simulink model "AP_DiffEQs"  (Simulink 8.4)
settings: Solver=ode45  StartTime=0.0  StopTime=10.0  RelTol=1e-3
settings Model: Creator=Monica  LastModifiedBy=Monica
settings DataIOCC: SignalLoggingSaveFormat=Dataset
settings OptimizationCC: ExpressionDepthLimit=128
settings DebuggingCC: UnderspecifiedInitializationDetection=Simplified  MergeDetectMultiDrivingBlocksExec=error  FcnCallInpInsideContextMsg=EnableAllAsError  StateNameClashWarn=none
settings GRTTargetCC: CombineOutputUpdateFcns=on  GRTInterface=off

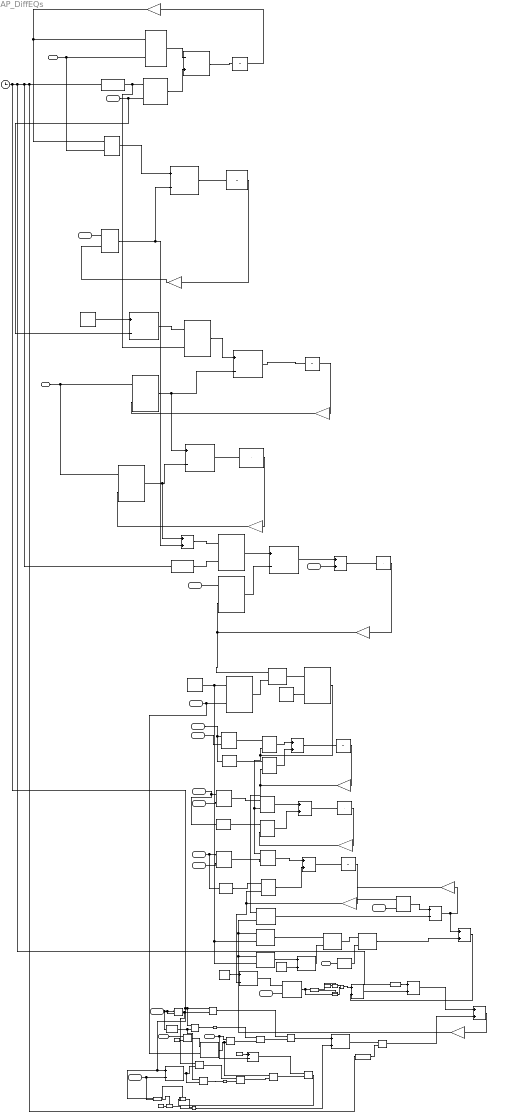
== system AP_DiffEQs ==
  note: 0
  note: false
  note: true
  note: t
  note: d
  note: Q_sub_2
  note: Q_sub_2
  note: Q_sub_1
  note: Q_sub_1
  note: Q_sub_1
  note: Q_sub_1
  note: -F_sub_01*(Q_sub_1/V)/(1+Q_sub_1/V)-x_sub_1*Q_sub_1+k_sub_12*Q_sub_2+EGP_0(1-x_sub_3)+f_sub_g+U_sub_m
  note: (U_sub_m1+U_sub_m2)*f_sub_m=U_sub_m
  note: f_sub_m
  note: t
  note: (U_sub_m1 + U_sub_m2)
  note: U_sub_m2
  note: (t-d)*(k_sub_m^2)*(exp((-k_sub_m)*(t-d)))*((CHO*5551)/w)*(1-p_sub_m)
  note: (1-p_sub_m)
  note: (1-p_sub_m)
  note: p_sub_m
  note: 1
  note: (t-d)*(k_sub_m^2)*(exp((-k_sub_m)*(t-d)))*((CHO*5551)/w)
  note: 0
  note: (t-d)*(k_sub_m^2)(*exp((-k_sub_m)*(t-d)))
  note: (t-d)*(k_sub_m^2)*(exp((-k_sub_m)*(t-d)))
  note: exp((-k_sub_m)*(t-d))
  note: (-k_sub_m)*(t-d)
  note: (t-d)
  note: -k_sub_m
  note: k_sub_m^2)
  note: (t-d)*(k_sub_m^2)
  note: (t-d)
  note: d
  note: t
  note: ((k_sub_m^2)*t)*exp(-k_sub_m*t)*((CHO*5551)/w)*p_sub_m
  note: exp(-k_sub_m*t)*((CHO*5551)/w)*p_sub_m
  note: ((k_sub_m^2)*t)
  note: ((CHO*5551)/w)*p_sub_m
  note: (CHO*5551)/w
  note: CHO*5551
  note: 5551
  note: CHO
  note: (k_sub_m^2*t)
  note: exp(-k_sub_m*t)
  note: -k_sub_m*t
  note: t
  note: -k_sub_m
  note: t
  note: k_sub_m^2
  note: k_sub_m
  note: k_sub_m
  note: -F_sub_01*(Q_sub_1/V)/(1+Q_sub_1/V)-x_sub_1*Q_sub_1+k_sub_12*Q_sub_2+EGP_0(1-x_sub_3)+f_sub_g
  note: -F_sub_01*(Q_sub_1/V)/(1+Q_sub_1/V)-x_sub_1*Q_sub_1+k_sub_12*Q_sub_2+EGP_0(1-x_sub_3)
  note: -F_sub_01*(Q_sub_1/V)/(1+Q_sub_1/V)-x_sub_1*Q_sub_1+k_sub_12*Q_sub_2
  note: EGP_0*(1-x_sub_3)
  note: 1
  note: EGP_0
  note: x_sub_3
  note: 1-x_sub_3
  note: -x_sub_1*Q_sub_1+k_sub_12*Q_sub_2
  note: x_sub_1*Q_sub_1
  note: k_sub_12*Q_sub_2
  note: -F_sub_01*(Q_sub_1/V)/(1+Q_sub_1/V)
  note: (Q_sub_1/V)/(1+Q_sub1/V)
  note: Q_sub_1/V + 1
  note: Q_sub_1/V
  note: x_sub_1
  note: V
  note: V
  note: Q_sub_1/V
  note: -F_sub_01
  note: F_sub_01
  note: x_sub_3
  note: -k_sub_a3*x_sub_3+k_sub_a3*S_sub_e*I_sub_p
  note: -k_sub_a3*x_sub_3
  note: k_sub_a3*S_sub_e*I_sub_p
  note: x_sub_3
  note: -k_sub_a3
  note: k_sub_a3*S_sub_e
  note: S_sub_e
  note: k_sub_a3
  note: k_sub_a3
  note: x_sub_2
  note: -k_sub_a2*x_sub_2+k_sub_a2*S_sub_d*I_sub_p
  note: -k_sub_a2*x_sub_2
  note: k_sub_a2*S_sub_d*I_sub_p
  note: k_sub_a2*S_sub_d
  note: I_sub_p
  note: -k_sub_a2
  note: k_sub_a2
  note: S_sub_d
  note: k_sub_a2
  note: x_sub_1
  note: -k_sub_a1
  note: -k_sub_a1*x_sub_1+k_sub_a1*S_sub_t*I_sub_p
  note: -k_sub_a1*x_sub_1
  note: I_sub_p
  note: k_sub_a1*S_sub_t*I_sub_p
  note: I_sub_p
  note: k_sub_a1
  note: S_sub_t
  note: k_sub_a1
  note: Q_sub_i/V_sub_i*w
  note: Q_sub_i
  note: w
  note: V_sub_i
  note: V_sub_i*w
  note: Q_sub_i
  note: ((Q_sub_is2*k_sub_is2+Q_sub_if2*k_sub_if)*I_sub_m)-Q_sub_i*k_sub_e+c_sub_i
  note: ((Q_sub_is2*k_sub_is2+Q_sub_if2*k_sub_if)*I_sub_m)-Q_subI*k_sub_e
  note: (Q_sub_is2*k_sub_is2+Q_sub_if2*k_sub_if)*I_sub_m
  note: Q_sub_i*k_sub_e
  note: I_sub_m
  note: Q_sub_is2*k_sub_is2+Q_sub_if2*k_sub_if
  note: Q_sub_is2*k_sub_is2
  note: Q_sub_if2*k_sub_if
  note: Q_sub_if1*k_sub_if-Q_sub_if2*k_sub_if
  note: Q_sub_if1*k_sub_if
  note: Q_sub_if2*k_sub_if
  note: Q_sub_if2
  note: k_sub_if
  note: Q_sub_if1
  note: (u_sub_i(t))*(1-p_sub_i)-Q_sub_i1f*k_sub_if
  note: Q_sub_if1*k_sub_if
  note: (u_sub_i(t))*(1-p_sub_i)
  note: u_sub_i(t)
  note: 1
  note: p_sub_i
  note: (1-p_sub_i)
  note: Q_sub_is1*k_sub_is1-Q_sub_is2*k_sub_is2
  note: Q_sub_is2*k_sub_is2
  note: Q_sub_is2
  note: Q_sub_is1*k_sub_is1
  note: k_sub_is1
  note: Q_sub_is1
  note: Q_sub_is1
  note: (u_sub_i(t)*p_sub_i)-(Q_sub_is1(t)*k_sub_is1)
  note: u_sub_i(t)*p_sub_i
  note: Q_sub_is1(t)*k_sub_is1
  p_sub_i : Inport
  "k_sub_is1 " : Inport  Port=2
  "k_sub_is2 " : Inport  Port=3
  k_sub_if : Inport  Port=4
  k_sub_e : Inport  Port=5
  c_sub_i : Inport  Port=6
  "w " : Inport  Port=7
  k_sub_a1 : Inport  Port=8
  S_sub_t : Inport  Port=9
  k_sub_a2 : Inport  Port=10
  S_sub_d : Inport  Port=11
  k_sub_a3 : Inport  Port=12
  S_sub_e : Inport  Port=13
  F_sub_01 : Inport  Port=14
  k_sub_12 : Inport  Port=15
  EGP_0 : Inport  Port=16
  k_sub_m : Inport  Port=17
  CHO : Inport  Port=18
  p_sub_m : Inport  Port=19
  d : Inport  Port=20
  " " : FunctionCaller  FunctionPrototype=u_sub_i = f(t)
  10^6 : Constant  Value=10^6
  Add{,1..5,8..10,13..14} (11 alike) : Sum
  Add{6..7,11..12} (4 alike) : Sum  Inputs=+-
  Clock : Clock
  Constant{,1..2,6} (4 alike) : Constant
  Constant3 : Constant  Value=0
  Constant4 : Constant  Value=5551
  Constant5 : Constant  Value=0
  Divide{,1..4} (5 alike) : Product  Inputs=*/
  Gain{,1..9} (10 alike) : Gain
  I_sub_m(t) : FunctionCaller  FunctionPrototype=I_sub_m = f(t)
  If : If  IfExpression=u1 >= 1
  If Action Subsystem : Subsystem  TreatAsAtomicUnit=on
  If Action Subsystem1 : Subsystem  TreatAsAtomicUnit=on
  If Action Subsystem2 : Subsystem  TreatAsAtomicUnit=on
  If Action Subsystem3 : Subsystem  TreatAsAtomicUnit=on
  Integrator{,1..7} (8 alike) : Integrator
  Math Function : Math  SaturateOnIntegerOverflow=on
  Math Function1 : Math  SaturateOnIntegerOverflow=on
  Merge : Merge
  Merge1 : Merge
  Product{,1..36} (37 alike) : Product
  Subtract : Sum  Inputs=-+
  Subtract{1..5} (5 alike) : Sum  Inputs=+-
  Subtract{6..10} (5 alike) : Sum  Inputs=-
  V_sub_i : Constant  Value=190
  f_sub_g : FunctionCaller  FunctionPrototype=f_sub_g = f(t)
  f_sub_m(t) : FunctionCaller  FunctionPrototype=f_sub_m = f(t)
  t-d : If  NumInputs=2  IfExpression=u1 > u2
  "u_sub_i(t) " : FunctionCaller  FunctionPrototype=u_sub_i = f(t)
  wires:
  Clock/1 -> Add11/1, t-d/1, Product26/1, Product25/1, f_sub_g/1, I_sub_m(t)/1, f_sub_m(t)/1, " "/1
  "k_sub_is1 "/1 -> Product2/2, Product/2
  " "/1 -> Product4/2, Product1/1
  p_sub_i/1 -> Subtract2/2, Product1/2
  Product/1 -> Subtract/1
  Product1/1 -> Subtract/2
  Subtract/1 -> Integrator/1
  Integrator/1 -> Gain/1
  Gain/1 -> Product2/1, Product/1
  Product2/1 -> Subtract1/1
  "k_sub_is2 "/1 -> Product3/1
  Product3/1 -> Add/2, Subtract1/2
  Subtract1/1 -> Integrator1/1
  Integrator1/1 -> Gain1/1
  Gain1/1 -> Product3/2
  Constant/1 -> Subtract2/1
  Subtract2/1 -> Product4/1
  k_sub_if/1 -> Product6/1, Product5/1
  Product5/1 -> Subtract3/2, Subtract4/1
  Product4/1 -> Subtract3/1
  Subtract3/1 -> Integrator2/1
  Integrator2/1 -> Gain2/1
  Gain2/1 -> Product5/2
  Product6/1 -> Add/1, Subtract4/2
  Subtract4/1 -> Integrator3/1
  Integrator3/1 -> Gain3/1
  Gain3/1 -> Product6/2
  Add/1 -> Product7/1
  I_sub_m(t)/1 -> Product7/2
  Product7/1 -> Subtract5/1
  k_sub_e/1 -> Product8/1
  Product8/1 -> Subtract5/2
  Subtract5/1 -> Add1/1
  c_sub_i/1 -> Add1/2
  Add1/1 -> Integrator4/1
  Integrator4/1 -> Gain4/1
  Gain4/1 -> Divide/1, Product8/2
  Product9/1 -> Divide/2
  V_sub_i/1 -> Divide1/2, Divide2/2, Product9/1
  "w "/1 -> Divide4/2, Product9/2
  Divide/1 -> Product10/1
  10^6/1 -> Product10/2
  k_sub_a1/1 -> Subtract6/1, Product11/1
  S_sub_t/1 -> Product11/2
  Product11/1 -> Product12/1
  Subtract6/1 -> Product13/1
  Product10/1 -> Product18/1, Product16/2, Product12/2
  Product12/1 -> Add2/1
  Product13/1 -> Add2/2
  Add2/1 -> Integrator5/1
  Integrator5/1 -> Gain5/1
  Gain5/1 -> Product13/2, Product20/1
  k_sub_a2/1 -> Subtract7/1, Product14/1
  S_sub_d/1 -> Product14/2
  Subtract7/1 -> Product15/1
  Product14/1 -> Product16/1
  Product16/1 -> Add3/1
  Product15/1 -> Add3/2
  Add3/1 -> Integrator6/1
  Integrator6/1 -> Gain6/1
  Gain6/1 -> Product15/2
  k_sub_a3/1 -> Subtract8/1, Product17/1
  S_sub_e/1 -> Product17/2
  Product17/1 -> Product18/2
  Subtract8/1 -> Product19/1
  Product18/1 -> Add4/1
  Product19/1 -> Add4/2
  Integrator7/1 -> Gain7/1
  Add4/1 -> Integrator7/1
  Gain7/1 -> Product19/2, Add7/2
  Divide2/1 -> Add5/1
  Constant1/1 -> Add5/2
  Add5/1 -> Divide3/2
  Divide1/1 -> Divide3/1
  Divide3/1 -> Product21/1
  F_sub_01/1 -> Subtract9/1
  Subtract9/1 -> Product21/2
  Product21/1 -> Add8/2
  Product20/1 -> Add6/2
  Product22/1 -> Add6/1
  k_sub_12/1 -> Product22/2
  Add6/1 -> Add8/1, Gain9/1
  Constant2/1 -> Add7/1
  Add7/1 -> Product23/1
  EGP_0/1 -> Product23/2
  Add8/1 -> Add9/2
  Add9/1 -> Add10/2
  Add10/1 -> Add14/1
  Product23/1 -> If Action Subsystem1/1(In1), If/1
  If/2 -> If Action Subsystem1/Action
  If/1 -> If Action Subsystem/Action
  Constant3/1 -> If Action Subsystem/1(In1)
  If Action Subsystem/1(Out1) -> Merge/1
  If Action Subsystem1/1(Out1) -> Merge/2
  Merge/1 -> Add9/1
  f_sub_g/1 -> Add10/1
  k_sub_m/1 -> Subtract10/1, Product24/2, Product24/1
  Product24/1 -> Product31/1, Product25/2
  Subtract10/1 -> Product32/1, Product26/2
  Product26/1 -> Math Function/1
  Math Function/1 -> Product27/1
  Product25/1 -> Product30/1
  Constant4/1 -> Product28/2
  CHO/1 -> Product28/1
  Product28/1 -> Divide4/1
  Divide4/1 -> Product34/1, Product29/2
  p_sub_m/1 -> Add12/2, Product29/1
  Product29/1 -> Product27/2
  Product27/1 -> Product30/2
  Product30/1 -> Add13/1
  d/1 -> t-d/2, Add11/2
  Add11/1 -> Product32/2, Product31/2
  Product31/1 -> Product33/1
  Product32/1 -> Math Function1/1
  Math Function1/1 -> Product33/2
  t-d/1 -> If Action Subsystem2/Action
  t-d/2 -> If Action Subsystem3/Action
  Constant5/1 -> If Action Subsystem3/1(In1)
  If Action Subsystem2/1(Out1) -> Merge1/1
  If Action Subsystem3/1(Out1) -> Merge1/2
  Merge1/1 -> Add13/2
  Product33/1 -> Product34/2
  Product34/1 -> Product35/2
  Constant6/1 -> Add12/1
  Add12/1 -> Product35/1
  Product35/1 -> If Action Subsystem2/1(In1)
  Add13/1 -> Product36/1
  f_sub_m(t)/1 -> Product36/2
  Product36/1 -> Add14/2
  Add14/1 -> Gain8/1
  Gain8/1 -> Product20/2, Divide1/1, Divide2/1
  Gain9/1 -> Product22/1

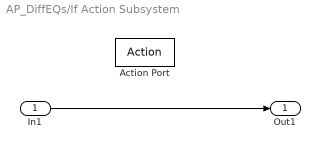
== system AP_DiffEQs/If Action Subsystem ==
  In1 : Inport
  Action Port : ActionPort  ActionType=then
  Out1 : Outport
  wires:
  In1/1 -> Out1/1

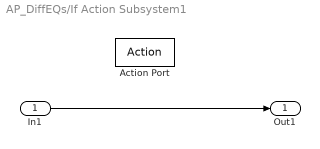
== system AP_DiffEQs/If Action Subsystem1 ==
  In1 : Inport
  Action Port : ActionPort  ActionType=else
  Out1 : Outport
  wires:
  In1/1 -> Out1/1

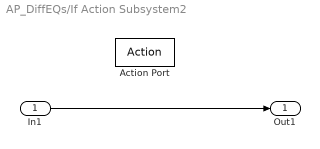
== system AP_DiffEQs/If Action Subsystem2 ==
  In1 : Inport
  Action Port : ActionPort  ActionType=then
  Out1 : Outport
  wires:
  In1/1 -> Out1/1

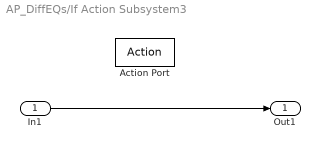
== system AP_DiffEQs/If Action Subsystem3 ==
  In1 : Inport
  Action Port : ActionPort  ActionType=else
  Out1 : Outport
  wires:
  In1/1 -> Out1/1
